simulink model "deployAMR_stateflow"  (R2024a)
settings: configuration reference "SharedConfig" (kept outside this file)
model workspace (MAT data in the model file):
  mdlWSDbList = ["C:\Users\matlab.cut\Desktop\AMR\canbus_files\tramontina_database_xsens.dbc" "tramontina_database_curtis.dbc"]
  mdlWSDbcList = ["C:\Users\rodri\Dev\Projects\External\Tramontina\atlas\interface_models\xsens.dbc" "tramontina_database_curtis.dbc"]
undefined symbols (not defined in the file): L, L_limited, magnitude, max_steering_angle_deg, num_of_wps, T, tstep, vehicle_wheelbase
libraries: simulink x3, simulink_extras x2
(part 1 of 2)
settings Model: DataDictionary=configuration_dictionary.sldd  Creator=rodri  LastModifiedBy=matlab.cut
settings ConfigSetRef: SourceName=SharedConfig

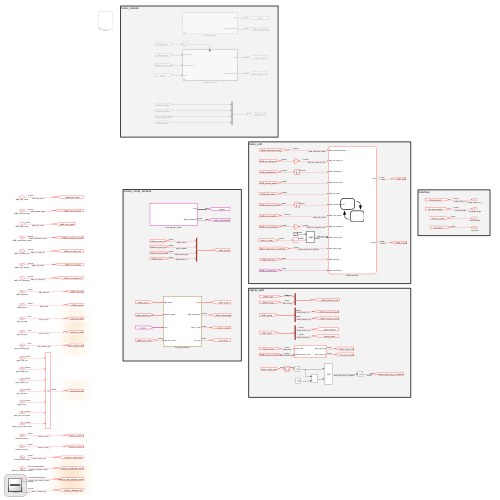
[thumbnail: Simulink's stored preview of the top-level diagram]
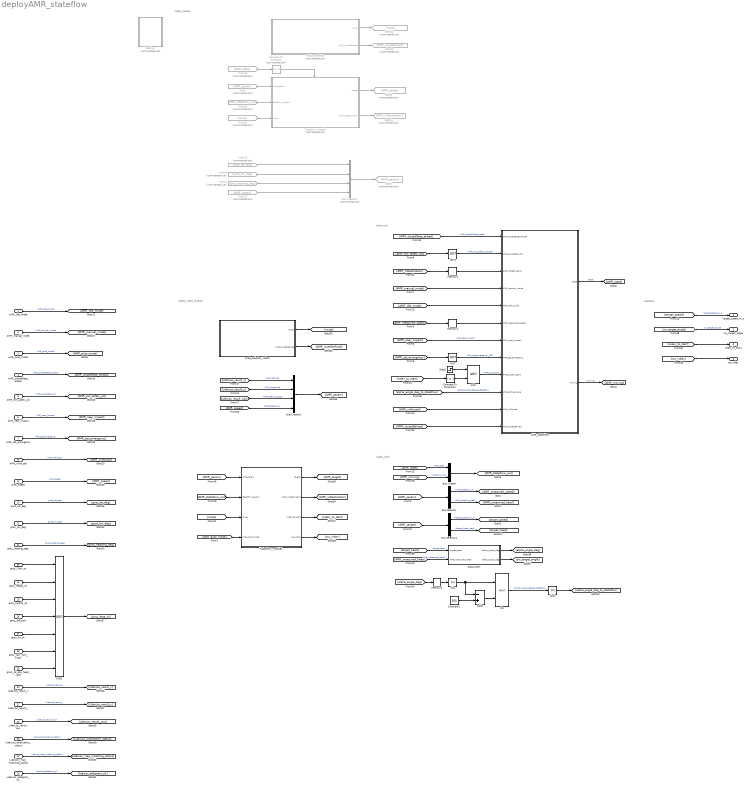
== system deployAMR_stateflow ==
  note: route_module
  note: brain_unit
  note: signal_split
  note: interface
  note: indoor_route_module
  AMR_idle_mode : Inport  OutDataTypeStr=boolean
  AMR_manual_mode : Inport  Port=2  OutDataTypeStr=boolean
  AMR_auto_mode : Inport  Port=3
  AMR_closedGate_ahead : Inport  Port=4  OutDataTypeStr=boolean
  AMR_ext_safety_plc : Inport  Port=5  OutDataTypeStr=boolean
  AMR_near_impact : Inport  Port=6  OutDataTypeStr=boolean
  AMR_set_emergency : Inport  Port=7  OutDataTypeStr=boolean
  AMR_withLoad : Inport  Port=8
  AMR_speed : Inport  Port=9
  gnss_lat_deg : Inport  Port=10  OutDataTypeStr=int32
  gnss_lon_deg : Inport  Port=11  OutDataTypeStr=int32
  gnss_heading_deg : Inport  Port=12  OutDataTypeStr=int32
  gnss_iToW_ok : Inport  Port=13
  gnss_height_ok : Inport  Port=14
  gnss_numSV_ok : Inport  Port=15
  gnss_diff_soln : Inport  Port=16
  gnss_fix_ok : Inport  Port=17
  gnss_carr_soln_fixed : Inport  Port=18
  gnss_rel_pos_head_valid : Inport  Port=19
  LidarLoc_result_x : Inport  Port=20
  LidarLoc_result_y : Inport  Port=21
  LidarLoc_result_yaw : Inport  Port=22
  LidarLoc_localization_status : Inport  Port=23  OutDataTypeStr=Enum: EnumLocalizationStatus
  LidarLoc_map_matching_status : Inport  Port=24  OutDataTypeStr=Enum: EnumMapMatchingStatus
  LidarLoc_telegram_ok : Inport  Port=25  OutDataTypeStr=boolean
  AMR_stateFlow : Stateflow chart  TreatAsAtomicUnit=on
  AND : Logic  AllPortsSameDT=off  OutDataTypeStr=boolean
  AND1 : Logic  Inputs=7  AllPortsSameDT=off  OutDataTypeStr=boolean
  Abs : Abs  SaturateOnIntegerOverflow=off
  Abs1 : Abs  SaturateOnIntegerOverflow=off
  Add1 : Sum  Inputs=-+
  Backup : Subsystem  Commented=on
  Bus Creator : BusCreator  Inputs=2
  Bus Creator1 : BusCreator  Inputs=4
  Bus Creator2 : BusCreator  Commented=on  Inputs=4
  Bus Selector : BusSelector  OutputSignals=AMR_speed_m_s,AMR_heading_deg
  Bus Selector1 : BusSelector  OutputSignals=target_speed_m_s,target_head_deg
  Compare To Constant : simulink/Logic and Bit Operations/Compare To Constant  Commented=on  relop===  const=2  OutDataTypeStr=boolean
  Compare To Constant1 : simulink/Logic and Bit Operations/Compare To Constant  relop=>=  const=1  OutDataTypeStr=boolean
  Constant2 : Constant  Value=360
  From : From  Commented=on  GotoTag=AMR_param
  From13 : From  Commented=on  GotoTag=AMR_state
  From14 : From  Commented=on  GotoTag=AMR_speed
  From18 : From  Commented=on  GotoTag=AMR_stateFlow_out
  From25 : From  Commented=on  GotoTag=route
  From29 : From  Commented=on  GotoTag=gnss_lat_deg
  From4 : From  Commented=on  GotoTag=gnss_lon_deg
  From5 : From  Commented=on  GotoTag=gnss_heading_deg
  Goto12 : Goto  Commented=on  GotoTag=route
  Goto13 : Goto  Commented=on  GotoTag=AMR_routeDefined
  Goto14 : Goto  Commented=on  GotoTag=AMR_inDestination
  Goto7 : Goto  Commented=on  GotoTag=AMR_param
  Goto8 : Goto  Commented=on  GotoTag=AMR_target
  Memory1 : Memory
  Memory2 : Memory
  Memory3 : Memory  InheritSampleTime=on
  Min : MinMax  Inputs=2
  NOT : Logic  Operator=NOT  IconShape=distinctive  AllPortsSameDT=off  OutDataTypeStr=boolean
  NOT1 : Logic  Operator=NOT  IconShape=distinctive  AllPortsSameDT=off  OutDataTypeStr=boolean
  Route_selector : Subsystem  Commented=on
  Step2 : Step  Time=10  SampleTime=0
  Subsystem : Subsystem
  Trajectory_module : Subsystem  Commented=on
  Trajectory_module1 : Subsystem
  route_selector_indoor : Subsystem
  target_speed_m_s : Outport
  sw_target_angle : Outport  Port=2
  index_to_start : Outport  Port=3
  wp_index : Outport  Port=4
  wires:
  AMR_stateFlow/2(moving) -> [AMR_moving]  "moving"
  AMR_stateFlow/1(state) -> [AMR_state]  "state"
  [AMR_ext_safety_plc] -> NOT1/1
  [AMR_manual_mode] -> AMR_stateFlow/4(AMR_manual_mode)
  [AMR_measured_speed] -> Memory1/1
  [AMR_near_impact] -> AMR_stateFlow/7(AMR_near_impact)  "AMR_near_impact"
  [AMR_set_emergency] -> NOT/1
  [AMR_withLoad] -> AMR_stateFlow/11(AMR_withLoad)
  [AMR_inDestination] -> Memory2/1
  [AMR_closedGate_ahead] -> AMR_stateFlow/1(AMR_closedGate_ahead)  "AMR_closedGate_ahead"
  From/1 -> Trajectory_module/1(AMR_param)
  Trajectory_module/1(target) -> Goto8/1
  From18/1 -> Trajectory_module/2(stateFlow_param)
  From13/1 -> Compare To Constant/1
  Compare To Constant/1 -> Trajectory_module/Enable
  [alpha_angle_deg_to_stateflow] -> AMR_stateFlow/10(AMR_alpha_angle)  "alpha_angle_deg_to_stateflow"
  Memory1/1 -> AMR_stateFlow/6(AMR_measured_speed)
  Route_selector/1(route) -> Goto12/1
  Route_selector/2(AMR_routeDefined) -> Goto13/1
  From25/1 -> Trajectory_module/3(route)
  [AMR_routeDefined] -> AMR_stateFlow/12(AMR_routeDefined)
  Trajectory_module/2(AMR_inDestination) -> Goto14/1
  Memory2/1 -> AMR_stateFlow/3(AMR_inDestination)
  AMR_closedGate_ahead/1 -> [AMR_closedGate_ahead]  "AMR_closedGate_ahead"
  AMR_manual_mode/1 -> [AMR_manual_mode]  "AMR_manual_mode"
  AMR_near_impact/1 -> [AMR_near_impact]  "AMR_near_impact"
  AMR_withLoad/1 -> [AMR_withLoad]  "AMR_withLoad"
  gnss_lat_deg/1 -> [gnss_lat_deg]  "gnss_lat_deg"
  gnss_lon_deg/1 -> [gnss_lon_deg]  "gnss_lon_deg"
  AMR_speed/1 -> [AMR_speed]  "AMR_speed"
  gnss_heading_deg/1 -> [gnss_heading_deg]  "gnss_heading_deg"
  AMR_set_emergency/1 -> [AMR_set_emergency]  "AMR_set_emergency"
  AMR_ext_safety_plc/1 -> [AMR_ext_safety_plc]  "AMR_ext_safety_plc"
  NOT1/1 -> AMR_stateFlow/2(AMR_ext_safety_plc)  "AMR_ext_safety_plc_NOT"
  NOT/1 -> AMR_stateFlow/8(AMR_set_emergency)  "AMR_set_emergency_NOT"
  Bus Creator/1 -> [AMR_stateFlow_out]
  [AMR_moving] -> Bus Creator/2  "AMR_moving"
  [AMR_state] -> Bus Creator/1  "AMR_state"
  Bus Selector/1 -> [AMR_measured_speed]  "<AMR_speed_m_s>"
  Bus Selector1/2 -> [target_head]  "<target_head_deg>"
  Bus Selector/2 -> [AMR_measured_head]  "<AMR_heading_deg>"
  Bus Selector1/1 -> [target_speed]  "<target_speed_m_s>"
  [AMR_param] -> Bus Selector/1
  [AMR_target] -> Bus Selector1/1
  [sw_target_angle] -> sw_target_angle/1  "sw_target_angle"
  [target_speed] -> target_speed_m_s/1  "target_speed_m_s"
  AMR_idle_mode/1 -> [AMR_idle_mode]  "AMR_idle_mode"
  [AMR_idle_mode] -> AMR_stateFlow/5(AMR_idle_mode)
  LidarLoc_result_x/1 -> [LidarLoc_result_x]  "LidarLoc_result_x"
  LidarLoc_result_y/1 -> [LidarLoc_result_y]  "LidarLoc_result_y"
  LidarLoc_result_yaw/1 -> [LidarLoc_result_yaw]  "LidarLoc_result_yaw"
  LidarLoc_localization_status/1 -> [LidarLoc_localization_status]  "licarLoc_licalization_status"
  LidarLoc_map_matching_status/1 -> [LidarLoc_map_matching_status]  "licarLoc_map_matching_status"
  LidarLoc_telegram_ok/1 -> [licarLoc_telegram_ok]  "licarLoc_telegram_ok"
  route_selector_indoor/2(AMR_routeDefined) -> [AMR_routeDefined]
  route_selector_indoor/1(route) -> [route]
  [route] -> Trajectory_module1/3(route)
  Trajectory_module1/1(target) -> [AMR_target]
  [AMR_param] -> Trajectory_module1/1(AMR_param)
  Bus Creator1/1 -> [AMR_param]
  [AMR_stateFlow_out] -> Trajectory_module1/2(stateFlow_param)
  Trajectory_module1/2(AMR_inDestination) -> [AMR_inDestination]
  [AMR_speed] -> Bus Creator1/4  "AMR_speed_m_s"
  [LidarLoc_result_yaw] -> Bus Creator1/3  "AMR_heading_deg"
  [LidarLoc_result_y] -> Bus Creator1/2  "AMR_Longitude"
  Bus Creator2/1 -> Goto7/1
  From29/1 -> Bus Creator2/1
  From4/1 -> Bus Creator2/2
  From5/1 -> Bus Creator2/3
  From14/1 -> Bus Creator2/4
  [LidarLoc_result_x] -> Bus Creator1/1  "AMR_Latitude"
  [AMR_measured_head] -> Subsystem/2(AMR_measured_head)  "AMR_measured_head"
  Subsystem/2(delta_angle_deg) -> [sw_target_angle]
  [target_head] -> Subsystem/1(target_head)  "target_head"
  [AMR_auto_mode] -> Trajectory_module1/4(AMR_auto_mode)
  AMR_auto_mode/1 -> [AMR_auto_mode]  "AMR_auto_mode"
  AND/1 -> AMR_stateFlow/9(AMR_system_start)  "AMR_syst_start"
  Step2/1 -> AND/1
  Compare To Constant1/1 -> AND/2
  [index_to_start] -> Compare To Constant1/1
  Trajectory_module1/3(index_to_start) -> [index_to_start]
  gnss_iToW_ok/1 -> AND1/1
  gnss_height_ok/1 -> AND1/2
  gnss_numSV_ok/1 -> AND1/3
  gnss_diff_soln/1 -> AND1/4
  AND1/1 -> [gnss_data_ok]
  gnss_fix_ok/1 -> AND1/5
  gnss_carr_soln_fixed/1 -> AND1/6
  gnss_rel_pos_head_valid/1 -> AND1/7
  Subsystem/1(alpha_angle_deg) -> [alpha_angle_deg]
  [index_to_start] -> index_to_start/1
  Trajectory_module1/4(wp_index) -> [wp_index]
  [wp_index] -> wp_index/1
  [alpha_angle_deg] -> Memory3/1
  Min/1 -> Abs1/1  "alpha_angle_deg_to_stateflow"
  Memory3/1 -> Abs/1
  Abs/1 -> Add1/1, Min/1
  Constant2/1 -> Add1/2
  Add1/1 -> Min/2
  Abs1/1 -> [alpha_angle_deg_to_stateflow]

== system deployAMR_stateflow/Backup ==
  Add : Sum  Inputs=+-
  Constant5 : Constant  Value=0
  GPS : Subsystem  Commented=on
  GPS_speed_measure : Subsystem  Commented=on
  Step : Step  Time=10  After=.000005  SampleTime=0
  Step1 : Step  Time=50  After=.000005  SampleTime=0
  wires:
  GPS_speed_measure/2(heading_deg) -> [agv_measured_heading]
  GPS/1(POS) -> [agv_pos]
  Constant5/1 -> GPS/1(dlat)
  Step1/1 -> Add/2
  Add/1 -> GPS/2(dlng)
  [agv_pos] -> GPS_speed_measure/1(GPS_POS)
  Step/1 -> Add/1
  GPS_speed_measure/1(speed_m_s) -> [agv_measured_speed]

== system deployAMR_stateflow/Route_selector ==
  Bus Creator4 : BusCreator  Inputs=2
  Constant : Constant
  Constant5 : Constant  Value=T.Latitude
  Constant9 : Constant  Value=T.Longitude
  route : Outport
  AMR_routeDefined : Outport  Port=2
  wires:
  Bus Creator4/1 -> route/1  "route"
  Constant9/1 -> Bus Creator4/2  "Longitude"
  Constant5/1 -> Bus Creator4/1  "Latitude"
  Constant/1 -> AMR_routeDefined/1

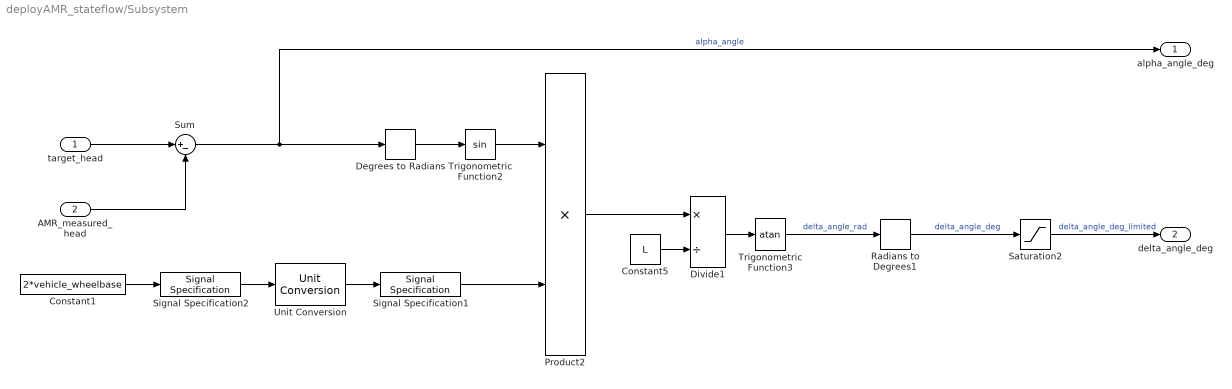
== system deployAMR_stateflow/Subsystem ==
  target_head : Inport
  AMR_measured_head : Inport  Port=2
  Constant1 : Constant  Value=2*vehicle_wheelbase
  Constant5 : Constant  Value=L
  Degrees to Radians : simulink_extras/Transformations/Degrees to Radians
  Divide1 : Product  Inputs=*/
  Product2 : Product
  Radians to Degrees1 : simulink_extras/Transformations/Radians to Degrees
  Saturation2 : Saturate  UpperLimit=max_steering_angle_deg  LowerLimit=-max_steering_angle_deg
  Signal Specification1 : SignalSpecification  Unit=m
  Signal Specification2 : SignalSpecification  Unit=mm
  Sum : Sum  Inputs=|+-
  Trigonometric Function2 : Trigonometry
  Trigonometric Function3 : Trigonometry  Operator=atan  ApproximationMethod=CORDIC
  Unit Conversion : UnitConversion
  alpha_angle_deg : Outport
  delta_angle_deg : Outport  Port=2
  wires:
  Degrees to Radians/1 -> Trigonometric Function2/1
  Constant1/1 -> Signal Specification2/1
  Product2/1 -> Divide1/1
  Radians to Degrees1/1 -> Saturation2/1  "delta_angle_deg"
  Sum/1 -> Degrees to Radians/1, alpha_angle_deg/1  "alpha_angle"
  Trigonometric Function2/1 -> Product2/1
  Constant5/1 -> Divide1/2
  Trigonometric Function3/1 -> Radians to Degrees1/1  "delta_angle_rad"
  Divide1/1 -> Trigonometric Function3/1
  target_head/1 -> Sum/1
  AMR_measured_head/1 -> Sum/2
  Saturation2/1 -> delta_angle_deg/1  "delta_angle_deg_limited"
  Unit Conversion/1 -> Signal Specification1/1
  Signal Specification2/1 -> Unit Conversion/1
  Signal Specification1/1 -> Product2/2

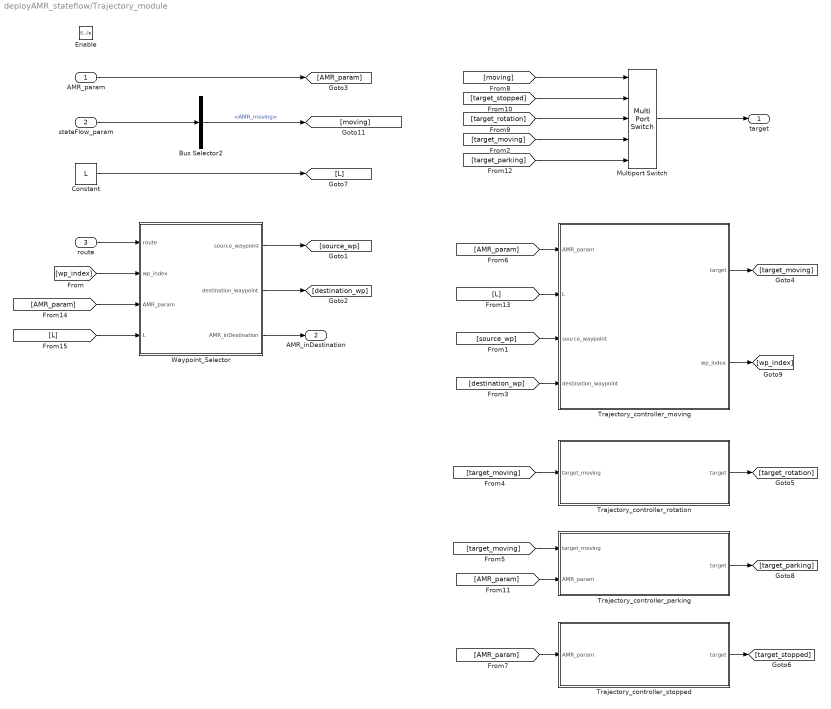
== system deployAMR_stateflow/Trajectory_module ==
  AMR_param : Inport
  stateFlow_param : Inport  Port=2
  route : Inport  Port=3
  Enable : EnablePort
  Bus Selector2 : BusSelector  OutputSignals=AMR_moving
  Constant : Constant  Value=L
  Multiport Switch : MultiPortSwitch  DataPortOrder=Zero-based contiguous  Inputs=4  zeroidx=on  SaturateOnIntegerOverflow=off  InputSameDT=off
  Trajectory_controller_moving : Subsystem
  Trajectory_controller_parking : Subsystem
  Trajectory_controller_rotation : Subsystem
  Trajectory_controller_stopped : Subsystem
  Waypoint_Selector : Subsystem
  target : Outport
  AMR_inDestination : Outport  Port=2
  wires:
  Trajectory_controller_moving/2(wp_index) -> [wp_index]
  [wp_index] -> Waypoint_Selector/2(wp_index)
  Trajectory_controller_moving/1(target) -> [target_moving]
  route/1 -> Waypoint_Selector/1(route)
  [L] -> Trajectory_controller_moving/2(L)
  Bus Selector2/1 -> [moving]  "<AMR_moving>"
  stateFlow_param/1 -> Bus Selector2/1
  [source_wp] -> Trajectory_controller_moving/3(source_waypoint)
  Waypoint_Selector/1(source_waypoint) -> [source_wp]
  Waypoint_Selector/2(destination_waypoint) -> [destination_wp]
  [destination_wp] -> Trajectory_controller_moving/4(destination_waypoint)
  AMR_param/1 -> [AMR_param]
  [AMR_param] -> Trajectory_controller_moving/1(AMR_param)
  Trajectory_controller_rotation/1(target) -> [target_rotation]
  Multiport Switch/1 -> target/1
  [moving] -> Multiport Switch/1
  [target_stopped] -> Multiport Switch/2
  [target_parking] -> Multiport Switch/5
  [target_moving] -> Multiport Switch/4
  [target_rotation] -> Multiport Switch/3
  [target_moving] -> Trajectory_controller_rotation/1(target_moving)
  [target_moving] -> Trajectory_controller_parking/1(target_moving)
  Trajectory_controller_parking/1(target) -> [target_parking]
  [AMR_param] -> Trajectory_controller_parking/2(AMR_param)
  [AMR_param] -> Trajectory_controller_stopped/1(AMR_param)
  Trajectory_controller_stopped/1(target) -> [target_stopped]
  Constant/1 -> [L]
  [AMR_param] -> Waypoint_Selector/3(AMR_param)
  [L] -> Waypoint_Selector/4(L)
  Waypoint_Selector/3(AMR_inDestination) -> AMR_inDestination/1

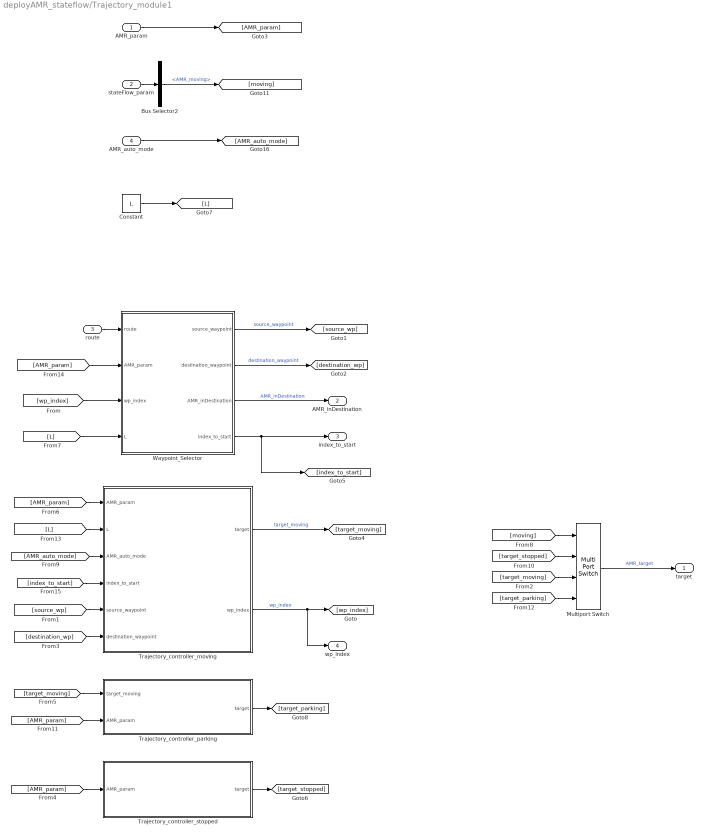
== system deployAMR_stateflow/Trajectory_module1 ==
  AMR_param : Inport
  stateFlow_param : Inport  Port=2
  route : Inport  Port=3
  AMR_auto_mode : Inport  Port=4
  Bus Selector2 : BusSelector  OutputSignals=AMR_moving
  Constant : Constant  Value=L
  Multiport Switch : MultiPortSwitch  DataPortOrder=Zero-based contiguous  zeroidx=on  SaturateOnIntegerOverflow=off  InputSameDT=off
  Trajectory_controller_moving : Subsystem
  Trajectory_controller_parking : Subsystem
  Trajectory_controller_stopped : Subsystem
  Waypoint_Selector : Subsystem
  target : Outport
  AMR_inDestination : Outport  Port=2
  index_to_start : Outport  Port=3
  wp_index : Outport  Port=4
  wires:
  Trajectory_controller_moving/2(wp_index) -> wp_index/1, [wp_index]  "wp_index"
  [wp_index] -> Waypoint_Selector/3(wp_index)
  Trajectory_controller_moving/1(target) -> [target_moving]  "target_moving"
  route/1 -> Waypoint_Selector/1(route)
  [L] -> Trajectory_controller_moving/2(L)
  Bus Selector2/1 -> [moving]  "<AMR_moving>"
  stateFlow_param/1 -> Bus Selector2/1
  [source_wp] -> Trajectory_controller_moving/5(source_waypoint)
  Waypoint_Selector/1(source_waypoint) -> [source_wp]  "source_waypoint"
  Waypoint_Selector/2(destination_waypoint) -> [destination_wp]  "destination_waypoint"
  [destination_wp] -> Trajectory_controller_moving/6(destination_waypoint)
  AMR_param/1 -> [AMR_param]
  [AMR_param] -> Trajectory_controller_moving/1(AMR_param)
  Multiport Switch/1 -> target/1  "AMR_target"
  [moving] -> Multiport Switch/1
  [target_stopped] -> Multiport Switch/2
  [target_moving] -> Trajectory_controller_parking/1(target_moving)
  Trajectory_controller_parking/1(target) -> [target_parking]
  [AMR_param] -> Trajectory_controller_parking/2(AMR_param)
  [AMR_param] -> Trajectory_controller_stopped/1(AMR_param)
  Trajectory_controller_stopped/1(target) -> [target_stopped]
  Constant/1 -> [L]
  [AMR_param] -> Waypoint_Selector/2(AMR_param)
  [L] -> Waypoint_Selector/4(L)
  Waypoint_Selector/3(AMR_inDestination) -> AMR_inDestination/1  "AMR_inDestination"
  [target_moving] -> Multiport Switch/3
  [target_parking] -> Multiport Switch/4
  AMR_auto_mode/1 -> [AMR_auto_mode]
  [AMR_auto_mode] -> Trajectory_controller_moving/3(AMR_auto_mode)
  [index_to_start] -> Trajectory_controller_moving/4(index_to_start)
  Waypoint_Selector/4(index_to_start) -> [index_to_start], index_to_start/1

== system deployAMR_stateflow/route_selector_indoor ==
  Bus Creator : BusCreator  Inputs=2
  Constant : Constant  Value=T.X
  Constant1 : Constant  Value=T.Y
  Constant2 : Constant
  route : Outport
  AMR_routeDefined : Outport  Port=2
  wires:
  Constant1/1 -> Bus Creator/2  "Y"
  Constant/1 -> Bus Creator/1  "X"
  Bus Creator/1 -> route/1  "route"
  Constant2/1 -> AMR_routeDefined/1

== system deployAMR_stateflow/Backup/GPS ==
  dlat : Inport
  dlng : Inport  Port=2
  Add : Sum  Inputs=|++
  Add1 : Sum  Inputs=|++
  Matrix Concatenate : Concatenate  Mode=Multidimensional array  ConcatenateDimension=2
  lat : Memory  InitialCondition=-29.272334
  lng : Memory  InitialCondition=-51.467679
  POS : Outport
  wires:
  lat/1 -> Add1/2, Matrix Concatenate/1
  Matrix Concatenate/1 -> POS/1
  dlat/1 -> Add1/1
  Add1/1 -> lat/1
  lng/1 -> Add/2, Matrix Concatenate/2
  Add/1 -> lng/1
  dlng/1 -> Add/1

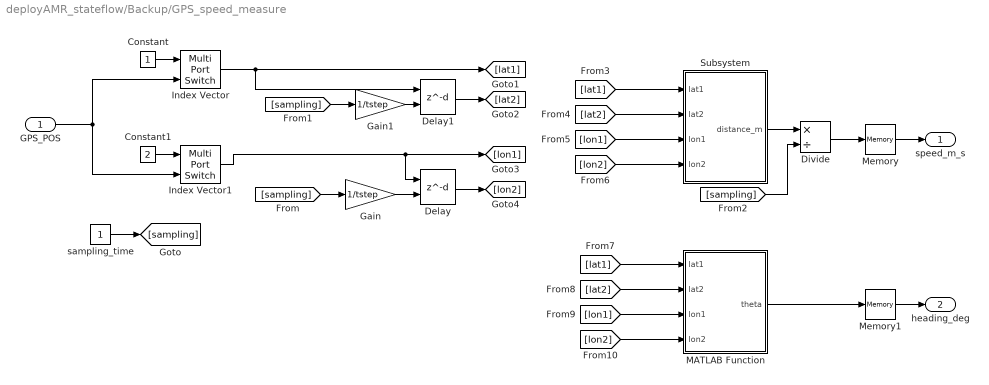
== system deployAMR_stateflow/Backup/GPS_speed_measure ==
  GPS_POS : Inport
  Constant : Constant
  Constant1 : Constant  Value=2
  Delay : Delay  DelayLengthSource=Input port  DelayLength=5/tstep  InitialCondition=-51.467679
      settings: InputPortMap=u0,p1
  Delay1 : Delay  DelayLengthSource=Input port  DelayLength=5/tstep  InitialCondition=-29.272334
      settings: InputPortMap=u0,p1
  Divide : Product  Inputs=*/
  Gain : Gain  Gain=1/tstep
  Gain1 : Gain  Gain=1/tstep
  Index Vector : MultiPortSwitch  Inputs=1  SaturateOnIntegerOverflow=off  InputSameDT=off
  Index Vector1 : MultiPortSwitch  Inputs=1  SaturateOnIntegerOverflow=off  InputSameDT=off
  MATLAB Function : MATLAB Function  TreatAsAtomicUnit=on
  Memory : Memory
  Memory1 : Memory
  Subsystem : Subsystem
  sampling_time : Constant
  speed_m_s : Outport
  heading_deg : Outport  Port=2
  wires:
  Subsystem/1(distance_m) -> Divide/1
  Memory/1 -> speed_m_s/1
  Divide/1 -> Memory/1
  Constant/1 -> Index Vector/1
  Constant1/1 -> Index Vector1/1
  Index Vector1/1 -> [lon1], Delay/1
  sampling_time/1 -> [sampling]
  Gain/1 -> Delay/2
  [sampling] -> Gain/1
  [sampling] -> Gain1/1
  Gain1/1 -> Delay1/2
  Index Vector/1 -> [lat1], Delay1/1
  GPS_POS/1 -> Index Vector/2, Index Vector1/2
  [sampling] -> Divide/2
  Memory1/1 -> heading_deg/1
  Delay1/1 -> [lat2]
  Delay/1 -> [lon2]
  [lat2] -> Subsystem/2(lat2)
  [lon1] -> Subsystem/3(lon1)
  [lon2] -> Subsystem/4(lon2)
  [lat1] -> Subsystem/1(lat1)
  [lon2] -> MATLAB Function/4(lon2)
  [lat1] -> MATLAB Function/1(lat1)
  [lon1] -> MATLAB Function/3(lon1)
  [lat2] -> MATLAB Function/2(lat2)
  MATLAB Function/1(theta) -> Memory1/1

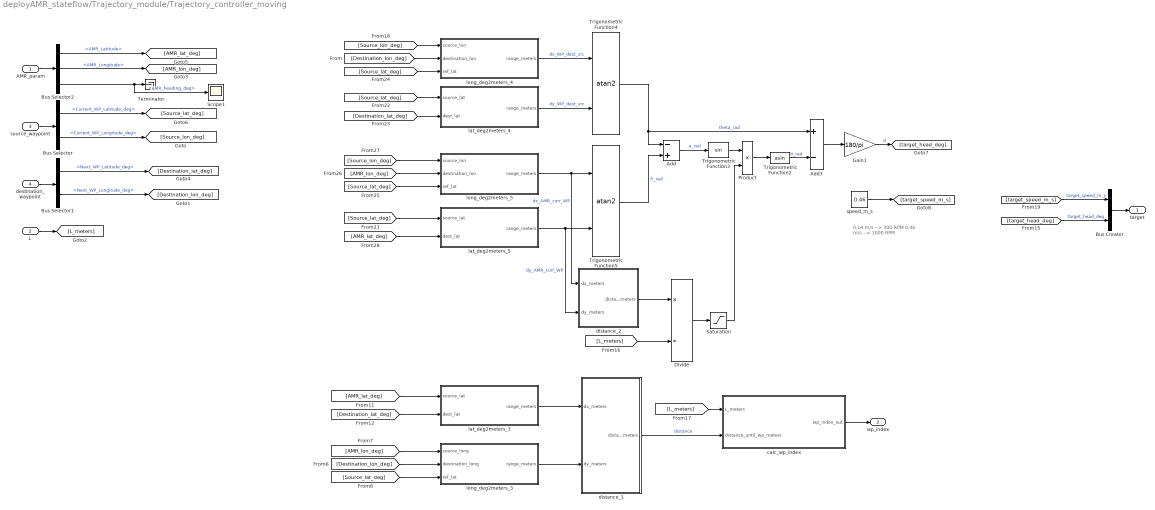
== system deployAMR_stateflow/Trajectory_module/Trajectory_controller_moving ==
  note: 0.14 m/s --> 300 RPM
      | 0.46 m/s --> 1000 RPM
  AMR_param : Inport
  L : Inport  Port=2
  source_waypoint : Inport  Port=3
  destination_waypoint : Inport  Port=4
  Add : Sum  Inputs=-+
  Add3 : Sum  Inputs=+-
  Bus Creator : BusCreator  Inputs=2
  Bus Selector : BusSelector  OutputSignals=Current_WP_Latitude_deg,Current_WP_Longitude_deg
  Bus Selector1 : BusSelector  OutputSignals=Next_WP_Latitude_deg,Next_WP_Longitude_deg
  Bus Selector2 : BusSelector  OutputSignals=AMR_Latitude,AMR_Longitude,AMR_heading_deg
  Divide : Product  Inputs=*/
  Gain1 : Gain  Gain=180/pi
  Product : Product
  Saturation : Saturate  UpperLimit=1  LowerLimit=0
  Scope1 : Scope
  Terminator : Terminator
  Trigonometric Function2 : Trigonometry  Operator=asin
  Trigonometric Function3 : Trigonometry
  Trigonometric Function4 : Trigonometry  Operator=atan2
  Trigonometric Function5 : Trigonometry  Operator=atan2
  calc_wp_index : Subsystem
  distance_1 : Subsystem  TreatAsAtomicUnit=on
  distance_2 : Subsystem  TreatAsAtomicUnit=on
  lat_deg2meters_3 : Subsystem  TreatAsAtomicUnit=on
  lat_deg2meters_4 : Subsystem  TreatAsAtomicUnit=on
  lat_deg2meters_5 : Subsystem  TreatAsAtomicUnit=on
  long_deg2meters_3 : Subsystem  TreatAsAtomicUnit=on
  long_deg2meters_4 : Subsystem  TreatAsAtomicUnit=on
  long_deg2meters_5 : Subsystem  TreatAsAtomicUnit=on
  speed_m_s : Constant  Value=0.46
  target : Outport
  wp_index : Outport  Port=2
  wires:
  distance_1/1(distance_meters) -> calc_wp_index/2(distance_until_wp_meters)  "distance"
  calc_wp_index/1(wp_index_out) -> wp_index/1
  [Destination_lon_deg] -> long_deg2meters_3/2(destination_long)
  [Source_lat_deg] -> long_deg2meters_3/3(ref_lat)
  Trigonometric Function4/1 -> Add3/1, Add/1  "theta_rad"
  [L_meters] -> Divide/2
  [L_meters] -> calc_wp_index/1(L_meters)
  source_waypoint/1 -> Bus Selector/1
  destination_waypoint/1 -> Bus Selector1/1
  AMR_param/1 -> Bus Selector2/1
  Bus Selector2/1 -> [AMR_lat_deg]  "<AMR_Latitude>"
  Bus Selector2/2 -> [AMR_lon_deg]  "<AMR_Longitude>"
  Bus Selector/1 -> [Source_lat_deg]  "<Current_WP_Latitude_deg>"
  Bus Selector1/2 -> [Destination_lon_deg]  "<Next_WP_Longitude_deg>"
  Bus Selector1/1 -> [Destination_lat_deg]  "<Next_WP_Latitude_deg>"
  Bus Selector/2 -> [Source_lon_deg]  "<Current_WP_Longitude_deg>"
  [AMR_lon_deg] -> long_deg2meters_3/1(source_long)
  L/1 -> [L_meters]
  [target_speed_m_s] -> Bus Creator/1  "target_speed_m_s"
  [target_head_deg] -> Bus Creator/2  "target_head_deg"
  Bus Creator/1 -> target/1
  Add/1 -> Trigonometric Function3/1  "a_rad"
  Trigonometric Function3/1 -> Product/1
  speed_m_s/1 -> [target_speed_m_s]
  Bus Selector2/3 -> Scope1/1, Terminator/1  "<AMR_heading_deg>"
  Gain1/1 -> [target_head_deg]  "d"
  distance_2/1(distance_meters) -> Divide/1
  [Destination_lat_deg] -> lat_deg2meters_3/2(dest_lat)
  [AMR_lat_deg] -> lat_deg2meters_3/1(source_lat)
  Trigonometric Function5/1 -> Add/2  "fi_rad"
  lat_deg2meters_3/1(range_meters) -> distance_1/1(dx_meters)
  long_deg2meters_3/1(range_meters) -> distance_1/2(dy_meters)
  long_deg2meters_4/1(range_meters) -> Trigonometric Function4/1  "dx_WP_dest_src"
  lat_deg2meters_4/1(range_meters) -> Trigonometric Function4/2  "dy_WP_dest_src"
  long_deg2meters_5/1(range_meters) -> distance_2/1(dx_meters), Trigonometric Function5/1  "dx_AMR_curr_WP"
  lat_deg2meters_5/1(range_meters) -> distance_2/2(dy_meters), Trigonometric Function5/2  "dy_AMR_curr_WP"
  Add3/1 -> Gain1/1
  [Source_lon_deg] -> long_deg2meters_5/1(source_lon)
  [Source_lat_deg] -> long_deg2meters_4/3(ref_lat)
  [Source_lat_deg] -> lat_deg2meters_4/1(source_lat)
  [Destination_lon_deg] -> long_deg2meters_4/2(destination_lon)
  [AMR_lon_deg] -> long_deg2meters_5/2(destination_lon)
  [Source_lat_deg] -> long_deg2meters_5/3(ref_lat)
  [Destination_lat_deg] -> lat_deg2meters_4/2(dest_lat)
  [Source_lat_deg] -> lat_deg2meters_5/1(source_lat)
  [Source_lon_deg] -> long_deg2meters_4/1(source_lon)
  [AMR_lat_deg] -> lat_deg2meters_5/2(dest_lat)
  Trigonometric Function2/1 -> Add3/2  "b_rad"
  Product/1 -> Trigonometric Function2/1
  Divide/1 -> Saturation/1
  Saturation/1 -> Product/2

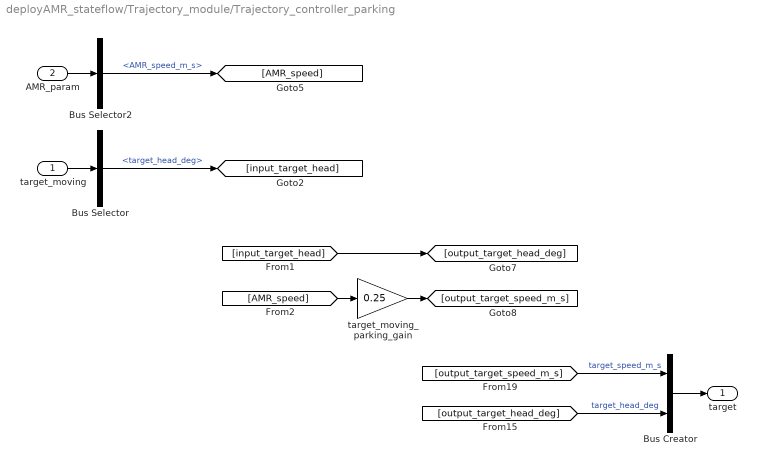
== system deployAMR_stateflow/Trajectory_module/Trajectory_controller_parking ==
  target_moving : Inport
  AMR_param : Inport  Port=2
  Bus Creator : BusCreator  Inputs=2
  Bus Selector : BusSelector  OutputSignals=target_head_deg
  Bus Selector2 : BusSelector  OutputSignals=AMR_speed_m_s
  target_moving_parking_gain : Gain  Gain=0.25
  target : Outport
  wires:
  [output_target_speed_m_s] -> Bus Creator/1  "target_speed_m_s"
  [output_target_head_deg] -> Bus Creator/2  "target_head_deg"
  Bus Creator/1 -> target/1
  [input_target_head] -> [output_target_head_deg]
  target_moving/1 -> Bus Selector/1
  AMR_param/1 -> Bus Selector2/1
  Bus Selector2/1 -> [AMR_speed]  "<AMR_speed_m_s>"
  Bus Selector/1 -> [input_target_head]  "<target_head_deg>"
  target_moving_parking_gain/1 -> [output_target_speed_m_s]
  [AMR_speed] -> target_moving_parking_gain/1

== system deployAMR_stateflow/Trajectory_module/Trajectory_controller_rotation ==
  target_moving : Inport
  Bus Creator : BusCreator  Inputs=2
  Bus Selector : BusSelector  OutputSignals=target_speed_m_s,target_head_deg
  target_moving_rotation_gain : Gain  Gain=0.5
  target : Outport
  wires:
  [output_target_speed_m_s] -> Bus Creator/1  "target_speed_m_s"
  [output_target_head_deg] -> Bus Creator/2  "target_head_deg"
  Bus Creator/1 -> target/1
  target_moving/1 -> Bus Selector/1
  Bus Selector/1 -> [input_target_speed]  "<target_speed_m_s>"
  Bus Selector/2 -> [input_target_head]  "<target_head_deg>"
  [input_target_speed] -> target_moving_rotation_gain/1
  [input_target_head] -> [output_target_head_deg]
  target_moving_rotation_gain/1 -> [output_target_speed_m_s]

== system deployAMR_stateflow/Trajectory_module/Trajectory_controller_stopped ==
  AMR_param : Inport
  Bus Creator : BusCreator  Inputs=2
  Bus Selector2 : BusSelector  OutputSignals=AMR_heading_deg
  Constant : Constant  Value=0
  target : Outport
  wires:
  [output_target_speed_m_s] -> Bus Creator/1  "target_speed_m_s"
  [output_target_head_deg] -> Bus Creator/2  "target_head_deg"
  Bus Creator/1 -> target/1
  [AMR_head] -> [output_target_head_deg]
  AMR_param/1 -> Bus Selector2/1
  Bus Selector2/1 -> [AMR_head]  "<AMR_heading_deg>"
  Constant/1 -> [output_target_speed_m_s]

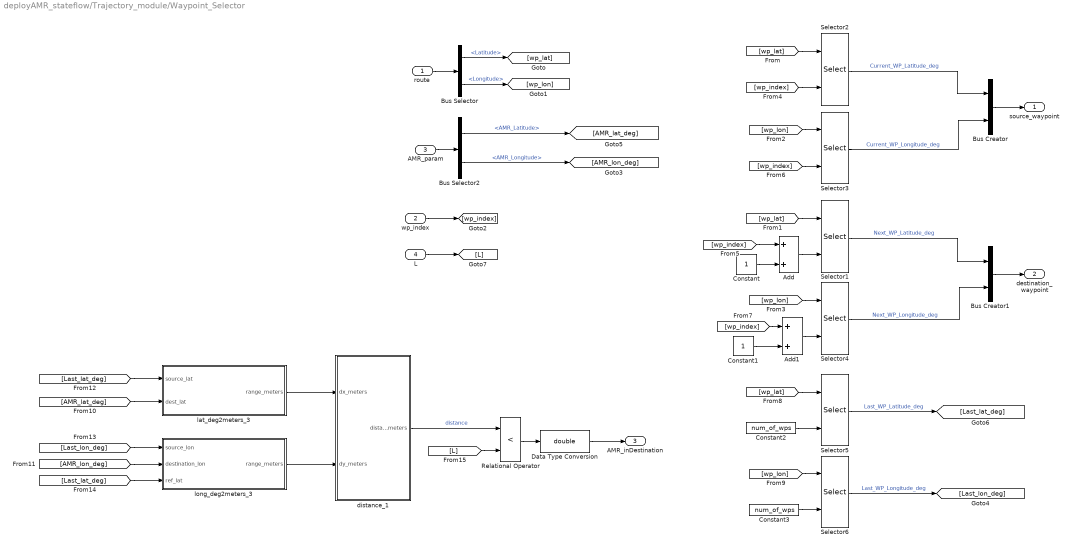
== system deployAMR_stateflow/Trajectory_module/Waypoint_Selector ==
  route : Inport
  wp_index : Inport  Port=2
  AMR_param : Inport  Port=3
  L : Inport  Port=4
  Add : Sum
  Add1 : Sum
  Bus Creator : BusCreator  Inputs=2
  Bus Creator1 : BusCreator  Inputs=2
  Bus Selector : BusSelector  OutputSignals=Latitude,Longitude
  Bus Selector2 : BusSelector  OutputSignals=AMR_Latitude,AMR_Longitude
  Constant : Constant
  Constant1 : Constant
  Constant2 : Constant  Value=num_of_wps
  Constant3 : Constant  Value=num_of_wps
  Data Type Conversion : DataTypeConversion  OutDataTypeStr=double  SaturateOnIntegerOverflow=off  RndMeth=Floor
  Relational Operator : RelationalOperator  Operator=<  OutDataTypeStr=boolean  RndMeth=Simplest  InputSameDT=off
  Selector{1..6} (6 alike) : Selector  InputPortWidth=num_of_wps  IndexOptions=Index vector (port)  Indices=[1 3]  OutputSizes=1
  distance_1 : Subsystem  TreatAsAtomicUnit=on
  lat_deg2meters_3 : Subsystem  TreatAsAtomicUnit=on
  long_deg2meters_3 : Subsystem  TreatAsAtomicUnit=on
  source_waypoint : Outport
  destination_waypoint : Outport  Port=2
  AMR_inDestination : Outport  Port=3
  wires:
  Selector2/1 -> Bus Creator/1  "Current_WP_Latitude_deg"
  Add/1 -> Selector1/2
  Constant/1 -> Add/2
  Constant1/1 -> Add1/2
  Add1/1 -> Selector4/2
  route/1 -> Bus Selector/1
  Bus Selector/1 -> [wp_lat]  "<Latitude>"
  Bus Selector/2 -> [wp_lon]  "<Longitude>"
  [wp_lat] -> Selector2/1
  [wp_lat] -> Selector1/1
  [wp_lon] -> Selector3/1
  [wp_lon] -> Selector4/1
  wp_index/1 -> [wp_index]
  [wp_index] -> Selector2/2
  [wp_index] -> Add/1
  [wp_index] -> Selector3/2
  [wp_index] -> Add1/1
  Bus Creator/1 -> source_waypoint/1
  Selector3/1 -> Bus Creator/2  "Current_WP_Longitude_deg"
  Selector4/1 -> Bus Creator1/2  "Next_WP_Longitude_deg"
  Selector1/1 -> Bus Creator1/1  "Next_WP_Latitude_deg"
  Bus Creator1/1 -> destination_waypoint/1
  Bus Selector2/1 -> [AMR_lat_deg]  "<AMR_Latitude>"
  AMR_param/1 -> Bus Selector2/1
  Bus Selector2/2 -> [AMR_lon_deg]  "<AMR_Longitude>"
  [wp_lat] -> Selector5/1
  [wp_lon] -> Selector6/1
  Constant3/1 -> Selector6/2
  Constant2/1 -> Selector5/2
  long_deg2meters_3/1(range_meters) -> distance_1/2(dy_meters)
  lat_deg2meters_3/1(range_meters) -> distance_1/1(dx_meters)
  Selector5/1 -> [Last_lat_deg]  "Last_WP_Latitude_deg"
  Selector6/1 -> [Last_lon_deg]  "Last_WP_Longitude_deg"
  [Last_lat_deg] -> lat_deg2meters_3/1(source_lat)
  [Last_lon_deg] -> long_deg2meters_3/1(source_lon)
  [Last_lat_deg] -> long_deg2meters_3/3(ref_lat)
  [AMR_lat_deg] -> lat_deg2meters_3/2(dest_lat)
  [AMR_lon_deg] -> long_deg2meters_3/2(destination_lon)
  Relational Operator/1 -> Data Type Conversion/1
  distance_1/1(distance_meters) -> Relational Operator/1  "distance"
  L/1 -> [L]
  [L] -> Relational Operator/2
  Data Type Conversion/1 -> AMR_inDestination/1

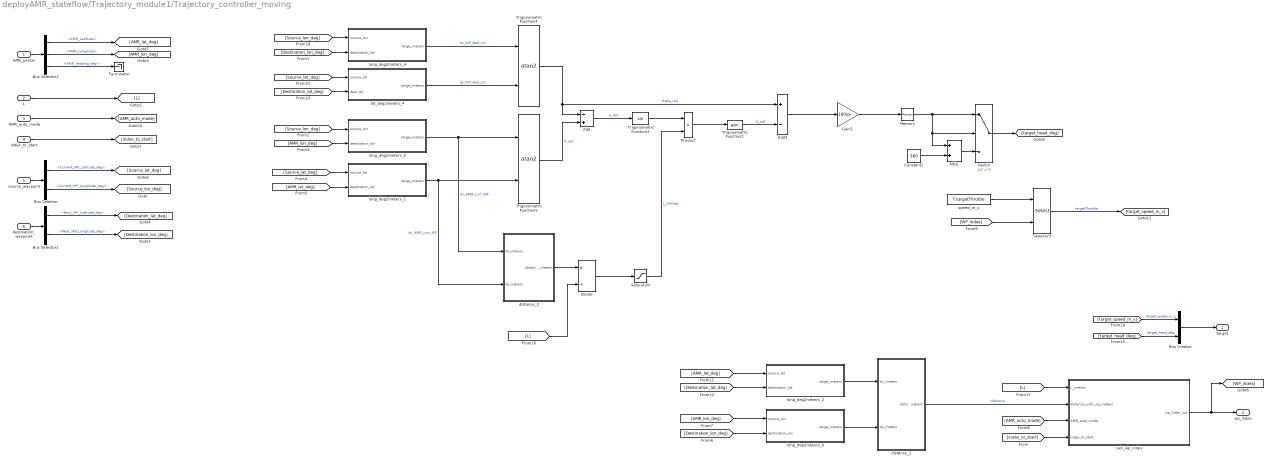
== system deployAMR_stateflow/Trajectory_module1/Trajectory_controller_moving ==
  AMR_param : Inport
  L : Inport  Port=2
  AMR_auto_mode : Inport  Port=3
  index_to_start : Inport  Port=4
  source_waypoint : Inport  Port=5
  destination_waypoint : Inport  Port=6
  Add : Sum  Inputs=-+
  Add1 : Sum
  Add3 : Sum  Inputs=+-
  Bus Creator : BusCreator  Inputs=2
  Bus Selector : BusSelector  OutputSignals=Current_WP_Latitude_deg,Current_WP_Longitude_deg
  Bus Selector1 : BusSelector  OutputSignals=Next_WP_Latitude_deg,Next_WP_Longitude_deg
  Bus Selector2 : BusSelector  OutputSignals=AMR_Latitude,AMR_Longitude,AMR_heading_deg
  Constant2 : Constant  Value=360
  Divide : Product  Inputs=*/
  Gain1 : Gain  Gain=180/pi
  Memory : Memory  InitialCondition=T.Yaw(1)  InheritSampleTime=on
  Product : Product
  Saturation : Saturate  UpperLimit=L_limited  LowerLimit=0
  Selector3 : Selector  InputPortWidth=num_of_wps  IndexOptions=Index vector (port)  Indices=[1 3]  OutputSizes=1
  Switch : Switch  Criteria=u2 > Threshold  SaturateOnIntegerOverflow=off  InputSameDT=off
  Terminator : Terminator
  Trigonometric Function2 : Trigonometry  Operator=asin
  Trigonometric Function3 : Trigonometry
  Trigonometric Function4 : Trigonometry  Operator=atan2
  Trigonometric Function5 : Trigonometry  Operator=atan2
  calc_wp_index : Subsystem
  distance_1 : Subsystem  TreatAsAtomicUnit=on
  distance_2 : Subsystem  TreatAsAtomicUnit=on
  lat_deg2meters_4 : Subsystem  TreatAsAtomicUnit=on
  long_deg2meters_1 : Subsystem  TreatAsAtomicUnit=on
  long_deg2meters_2 : Subsystem  TreatAsAtomicUnit=on
  long_deg2meters_4 : Subsystem  TreatAsAtomicUnit=on
  long_deg2meters_5 : Subsystem  TreatAsAtomicUnit=on
  long_deg2meters_6 : Subsystem  TreatAsAtomicUnit=on
  speed_m_s : Constant  Value=T.targetThrottle
  target : Outport
  wp_index : Outport  Port=2
  wires:
  [Source_lon_deg] -> long_deg2meters_5/1(source_lon)
  Add/1 -> Trigonometric Function3/1  "a_rad"
  [Destination_lat_deg] -> lat_deg2meters_4/2(dest_lat)
  Switch/1 -> [target_head_deg]
  distance_2/1(distance_meters) -> Divide/1
  Saturation/1 -> Product/2  "L_limited"
  Add1/1 -> Switch/3
  Product/1 -> Trigonometric Function2/1
  [AMR_lon_deg] -> long_deg2meters_5/2(destination_lon)
  Bus Creator/1 -> target/1
  destination_waypoint/1 -> Bus Selector1/1
  Add3/1 -> Gain1/1
  long_deg2meters_5/1(range_meters) -> Trigonometric Function5/1, distance_2/1(dx_meters)  "dx_AMR_curr_WP"
  [L] -> Divide/2
  AMR_param/1 -> Bus Selector2/1
  [Source_lon_deg] -> long_deg2meters_4/1(source_lon)
  lat_deg2meters_4/1(range_meters) -> Trigonometric Function4/2  "dy_WP_dest_src"
  [Destination_lat_deg] -> long_deg2meters_2/2(destination_lat)
  [Source_lat_deg] -> lat_deg2meters_4/1(source_lat)
  [AMR_lat_deg] -> long_deg2meters_2/1(source_lat)
  Trigonometric Function3/1 -> Product/1
  L/1 -> [L]
  Bus Selector2/3 -> Terminator/1  "<AMR_heading_deg>"
  long_deg2meters_2/1(range_meters) -> distance_1/1(dx_meters)
  [target_head_deg] -> Bus Creator/2  "target_head_deg"
  [Destination_lon_deg] -> long_deg2meters_6/2(destination_lon)
  Trigonometric Function5/1 -> Add/2  "fi_rad"
  Bus Selector2/1 -> [AMR_lat_deg]  "<AMR_Latitude>"
  Divide/1 -> Saturation/1
  Bus Selector2/2 -> [AMR_lon_deg]  "<AMR_Longitude>"
  Bus Selector/1 -> [Source_lat_deg]  "<Current_WP_Latitude_deg>"
  long_deg2meters_4/1(range_meters) -> Trigonometric Function4/1  "dx_WP_dest_src"
  [Destination_lon_deg] -> long_deg2meters_4/2(destination_lon)
  [Source_lat_deg] -> long_deg2meters_1/1(source_lat)
  [target_speed_m_s] -> Bus Creator/1  "target_speed_m_s"
  [AMR_lon_deg] -> long_deg2meters_6/1(source_lon)
  [AMR_lat_deg] -> long_deg2meters_1/2(destination_lat)
  Bus Selector1/1 -> [Destination_lat_deg]  "<Next_WP_Latitude_deg>"
  source_waypoint/1 -> Bus Selector/1
  Trigonometric Function4/1 -> Add3/1, Add/1  "theta_rad"
  Bus Selector1/2 -> [Destination_lon_deg]  "<Next_WP_Longitude_deg>"
  [L] -> calc_wp_index/1(L_meters)
  long_deg2meters_1/1(range_meters) -> Trigonometric Function5/2, distance_2/2(dy_meters)  "dy_AMR_curr_WP"
  Trigonometric Function2/1 -> Add3/2  "b_rad"
  long_deg2meters_6/1(range_meters) -> distance_1/2(dy_meters)
  Bus Selector/2 -> [Source_lon_deg]  "<Current_WP_Longitude_deg>"
  Constant2/1 -> Add1/2
  Gain1/1 -> Memory/1
  [AMR_auto_mode] -> calc_wp_index/3(AMR_auto_mode)
  [index_to_start] -> calc_wp_index/4(index_to_start)
  index_to_start/1 -> [index_to_start]
  AMR_auto_mode/1 -> [AMR_auto_mode]
  distance_1/1(distance_meters) -> calc_wp_index/2(distance_until_wp_meters)  "distance"
  [WP_index] -> Selector3/2
  Selector3/1 -> [target_speed_m_s]  "targetThrottle"
  speed_m_s/1 -> Selector3/1
  calc_wp_index/1(wp_index_out) -> [WP_index], wp_index/1
  Memory/1 -> Add1/1, Switch/2, Switch/1

== system deployAMR_stateflow/Trajectory_module1/Trajectory_controller_parking ==
  target_moving : Inport
  AMR_param : Inport  Port=2
  Bus Creator : BusCreator  Inputs=2
  Bus Selector : BusSelector  OutputSignals=target_head_deg
  Bus Selector2 : BusSelector  OutputSignals=AMR_speed_m_s
  Gain : Gain  Gain=0
  target : Outport
  wires:
  [output_target_speed_m_s] -> Bus Creator/1  "target_speed_m_s"
  [output_target_head_deg] -> Bus Creator/2  "target_head_deg"
  Bus Creator/1 -> target/1
  [input_target_head] -> [output_target_head_deg]
  target_moving/1 -> Bus Selector/1
  AMR_param/1 -> Bus Selector2/1
  Bus Selector2/1 -> [AMR_speed]  "<AMR_speed_m_s>"
  Bus Selector/1 -> [input_target_head]  "<target_head_deg>"
  Gain/1 -> [output_target_speed_m_s]
  [AMR_speed] -> Gain/1

== system deployAMR_stateflow/Trajectory_module1/Trajectory_controller_stopped ==
  AMR_param : Inport
  Bus Creator : BusCreator  Inputs=2
  Bus Selector2 : BusSelector  OutputSignals=AMR_heading_deg
  Constant : Constant  Value=0
  target : Outport
  wires:
  [output_target_speed_m_s] -> Bus Creator/1  "target_speed_m_s"
  [output_target_head_deg] -> Bus Creator/2  "target_head_deg"
  Bus Creator/1 -> target/1
  [AMR_head] -> [output_target_head_deg]
  AMR_param/1 -> Bus Selector2/1
  Bus Selector2/1 -> [AMR_head]  "<AMR_heading_deg>"
  Constant/1 -> [output_target_speed_m_s]

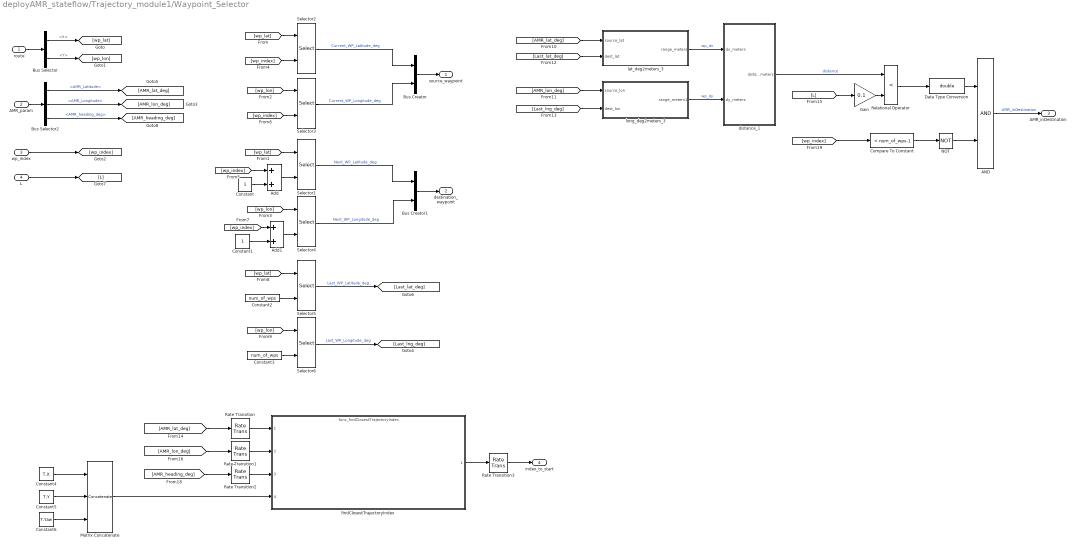
== system deployAMR_stateflow/Trajectory_module1/Waypoint_Selector ==
  route : Inport
  AMR_param : Inport  Port=2
  wp_index : Inport  Port=3
  L : Inport  Port=4
  AND : Logic  AllPortsSameDT=off  OutDataTypeStr=boolean
  Add : Sum
  Add1 : Sum
  Bus Creator : BusCreator  Inputs=2
  Bus Creator1 : BusCreator  Inputs=2
  Bus Selector : BusSelector  OutputSignals=X,Y
  Bus Selector2 : BusSelector  OutputSignals=AMR_Latitude,AMR_Longitude,AMR_heading_deg
  Compare To Constant : simulink/Logic and Bit Operations/Compare To Constant  relop=<  const=num_of_wps-1  OutDataTypeStr=boolean
  Constant : Constant
  Constant1 : Constant
  Constant2 : Constant  Value=num_of_wps
  Constant3 : Constant  Value=num_of_wps
  Constant4 : Constant  Value=T.X
  Constant5 : Constant  Value=T.Y
  Constant6 : Constant  Value=T.Yaw
  Data Type Conversion : DataTypeConversion  OutDataTypeStr=double  SaturateOnIntegerOverflow=off  RndMeth=Floor
  Gain : Gain  Gain=0.1
  Matrix Concatenate : Concatenate  NumInputs=3  Mode=Multidimensional array  ConcatenateDimension=2
  NOT : Logic  Operator=NOT  IconShape=distinctive  AllPortsSameDT=off  OutDataTypeStr=boolean
  Rate Transition{,1..3} (4 alike) : RateTransition
  Relational Operator : RelationalOperator  Operator=<  OutDataTypeStr=boolean  RndMeth=Simplest  InputSameDT=off
  Selector{1..6} (6 alike) : Selector  InputPortWidth=num_of_wps  IndexOptions=Index vector (port)  Indices=[1 3]  OutputSizes=1
  distance_1 : Subsystem  TreatAsAtomicUnit=on
  findClosestTrajectoryIndex : ModelReference  ModelNameDialog=func_findClosestTrajectoryIndex.slx  SimulationMode=Normal  ModelReferenceVersion=1.242
  lat_deg2meters_3 : Subsystem  TreatAsAtomicUnit=on
  long_deg2meters_3 : Subsystem  TreatAsAtomicUnit=on
  source_waypoint : Outport
  destination_waypoint : Outport  Port=2
  AMR_inDestination : Outport  Port=3
  index_to_start : Outport  Port=4
  wires:
  Selector2/1 -> Bus Creator/1  "Current_WP_Latitude_deg"
  Add/1 -> Selector1/2
  Constant/1 -> Add/2
  Constant1/1 -> Add1/2
  Add1/1 -> Selector4/2
  route/1 -> Bus Selector/1
  Bus Selector/1 -> [wp_lat]  "<X>"
  Bus Selector/2 -> [wp_lon]  "<Y>"
  [wp_lat] -> Selector2/1
  [wp_lat] -> Selector1/1
  [wp_lon] -> Selector3/1
  [wp_lon] -> Selector4/1
  wp_index/1 -> [wp_index]
  [wp_index] -> Selector2/2
  [wp_index] -> Add/1
  [wp_index] -> Selector3/2
  [wp_index] -> Add1/1
  Bus Creator/1 -> source_waypoint/1
  Selector3/1 -> Bus Creator/2  "Current_WP_Longitude_deg"
  Selector4/1 -> Bus Creator1/2  "Next_WP_Longitude_deg"
  Selector1/1 -> Bus Creator1/1  "Next_WP_Latitude_deg"
  Bus Creator1/1 -> destination_waypoint/1
  Bus Selector2/1 -> [AMR_lat_deg]  "<AMR_Latitude>"
  AMR_param/1 -> Bus Selector2/1
  Bus Selector2/2 -> [AMR_lon_deg]  "<AMR_Longitude>"
  [wp_lat] -> Selector5/1
  [wp_lon] -> Selector6/1
  Constant3/1 -> Selector6/2
  Constant2/1 -> Selector5/2
  long_deg2meters_3/1(range_meters1) -> distance_1/2(dy_meters)  "wp_dy"
  lat_deg2meters_3/1(range_meters) -> distance_1/1(dx_meters)  "wp_dx"
  Selector5/1 -> [Last_lat_deg]  "Last_WP_Latitude_deg"
  Selector6/1 -> [Last_lng_deg]  "Last_WP_Longitude_deg"
  [AMR_lat_deg] -> lat_deg2meters_3/1(source_lat)
  Relational Operator/1 -> Data Type Conversion/1
  distance_1/1(distance_meters) -> Relational Operator/1  "distance"
  L/1 -> [L]
  [L] -> Gain/1
  Data Type Conversion/1 -> AND/1
  [Last_lat_deg] -> lat_deg2meters_3/2(dest_lat)
  [AMR_lon_deg] -> long_deg2meters_3/1(source_lon)
  [Last_lng_deg] -> long_deg2meters_3/2(dest_lon)
  Matrix Concatenate/1 -> findClosestTrajectoryIndex/4
  [AMR_heading_deg] -> Rate Transition2/1
  [AMR_lon_deg] -> Rate Transition1/1
  Constant6/1 -> Matrix Concatenate/3
  Constant4/1 -> Matrix Concatenate/1
  [AMR_lat_deg] -> Rate Transition/1
  Constant5/1 -> Matrix Concatenate/2
  Bus Selector2/3 -> [AMR_heading_deg]  "<AMR_heading_deg>"
  findClosestTrajectoryIndex/1 -> Rate Transition3/1
  Rate Transition/1 -> findClosestTrajectoryIndex/1
  Rate Transition1/1 -> findClosestTrajectoryIndex/2
  Rate Transition2/1 -> findClosestTrajectoryIndex/3
  Rate Transition3/1 -> index_to_start/1
  [wp_index] -> Compare To Constant/1
  Compare To Constant/1 -> NOT/1
  NOT/1 -> AND/2
  AND/1 -> AMR_inDestination/1  "AMR_inDestination"
  Gain/1 -> Relational Operator/2

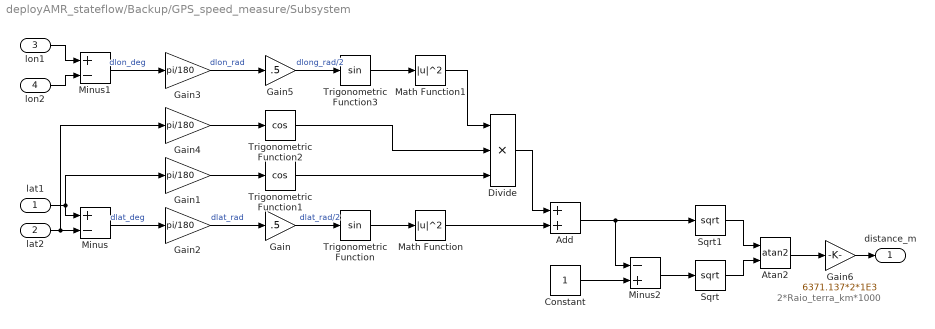
== system deployAMR_stateflow/Backup/GPS_speed_measure/Subsystem ==
  note: 2*Raio_terra_km*1000
  lat1 : Inport
  lat2 : Inport  Port=2
  lon1 : Inport  Port=3
  lon2 : Inport  Port=4
  Add : Sum
  Atan2 : Trigonometry  Operator=atan2
  Constant : Constant
  Divide : Product  Inputs=***
  Gain : Gain  Gain=.5
  Gain{1..4} (4 alike) : Gain  Gain=pi/180
  Gain5 : Gain  Gain=.5
  Gain6 : Gain  Gain=6371.137*2*1E3
  Math Function : Math  Operator=magnitude^2
  Math Function1 : Math  Operator=magnitude^2
  Minus : Sum  Inputs=+-
  Minus1 : Sum  Inputs=+-
  Minus2 : Sum  Inputs=-+
  Sqrt : Sqrt
  Sqrt1 : Sqrt
  Trigonometric Function : Trigonometry
  Trigonometric Function1 : Trigonometry  Operator=cos
  Trigonometric Function2 : Trigonometry  Operator=cos
  Trigonometric Function3 : Trigonometry
  distance_m : Outport
  wires:
  Minus/1 -> Gain2/1  "dlat_deg"
  Minus1/1 -> Gain3/1  "dlon_deg"
  lat2/1 -> Gain4/1, Minus/2
  lat1/1 -> Gain1/1, Minus/1
  lon1/1 -> Minus1/1
  lon2/1 -> Minus1/2
  Gain2/1 -> Gain/1  "dlat_rad"
  Gain/1 -> Trigonometric Function/1  "dlat_rad/2"
  Trigonometric Function/1 -> Math Function/1
  Math Function/1 -> Add/2
  Gain1/1 -> Trigonometric Function1/1
  Gain4/1 -> Trigonometric Function2/1
  Divide/1 -> Add/1
  Trigonometric Function3/1 -> Math Function1/1
  Gain5/1 -> Trigonometric Function3/1  "dlong_rad/2"
  Gain3/1 -> Gain5/1  "dlon_rad"
  Trigonometric Function1/1 -> Divide/3
  Trigonometric Function2/1 -> Divide/2
  Math Function1/1 -> Divide/1
  Add/1 -> Minus2/1, Sqrt1/1
  Minus2/1 -> Sqrt/1
  Atan2/1 -> Gain6/1
  Gain6/1 -> distance_m/1
  Constant/1 -> Minus2/2
  Sqrt1/1 -> Atan2/1
  Sqrt/1 -> Atan2/2

== system deployAMR_stateflow/Trajectory_module/Trajectory_controller_moving/calc_wp_index ==
  L_meters : Inport
  distance_until_wp_meters : Inport  Port=2
  Add : Sum
  Constant : Constant
  Data Type Conversion : DataTypeConversion  OutDataTypeStr=double  SaturateOnIntegerOverflow=off  RndMeth=Floor
  Memory : Memory  InitialCondition=1
  Relational Operator : RelationalOperator  Operator=>  OutDataTypeStr=boolean  RndMeth=Simplest  InputSameDT=off
  Saturation : Saturate  UpperLimit=num_of_wps-1  LowerLimit=1
  Scope3 : Scope
  Switch : Switch  Criteria=u2 > Threshold  Threshold=.5  SaturateOnIntegerOverflow=off  InputSameDT=off
  wp_index_out : Outport
  wires:
  distance_until_wp_meters/1 -> Relational Operator/1
  L_meters/1 -> Relational Operator/2
  Relational Operator/1 -> Data Type Conversion/1
  Data Type Conversion/1 -> Switch/2
  Switch/1 -> Memory/1
  Add/1 -> Switch/3
  Constant/1 -> Add/1
  [WP_index] -> wp_index_out/1, Scope3/1
  [WP_index] -> Switch/1
  [WP_index] -> Add/2
  Saturation/1 -> [WP_index]
  Memory/1 -> Saturation/1

== system deployAMR_stateflow/Trajectory_module/Trajectory_controller_moving/distance_1 ==
  dx_meters : Inport
  dy_meters : Inport  Port=2
  Add : Sum
  Divide1 : Product  Inputs=**
  Divide2 : Product  Inputs=**
  Sqrt : Sqrt
  distance_meters : Outport
  wires:
  dx_meters/1 -> Divide1/2, Divide1/1
  Divide1/1 -> Add/1
  Add/1 -> Sqrt/1
  dy_meters/1 -> Divide2/2, Divide2/1
  Divide2/1 -> Add/2
  Sqrt/1 -> distance_meters/1

== system deployAMR_stateflow/Trajectory_module/Trajectory_controller_moving/distance_2 ==
  dx_meters : Inport
  dy_meters : Inport  Port=2
  Add : Sum
  Divide1 : Product  Inputs=**
  Divide2 : Product  Inputs=**
  Sqrt : Sqrt
  distance_meters : Outport
  wires:
  dx_meters/1 -> Divide1/2, Divide1/1
  Divide1/1 -> Add/1
  Add/1 -> Sqrt/1
  dy_meters/1 -> Divide2/2, Divide2/1
  Divide2/1 -> Add/2
  Sqrt/1 -> distance_meters/1

== system deployAMR_stateflow/Trajectory_module/Trajectory_controller_moving/lat_deg2meters_3 ==
  source_lat : Inport
  dest_lat : Inport  Port=2
  Add : Sum  Inputs=+-
  deg2meters : Gain  Gain=111195
  range_meters : Outport
  wires:
  Add/1 -> deg2meters/1
  deg2meters/1 -> range_meters/1
  dest_lat/1 -> Add/1
  source_lat/1 -> Add/2

== system deployAMR_stateflow/Trajectory_module/Trajectory_controller_moving/lat_deg2meters_4 ==
  source_lat : Inport
  dest_lat : Inport  Port=2
  Add : Sum  Inputs=+-
  deg2meters : Gain  Gain=111195
  range_meters : Outport
  wires:
  Add/1 -> deg2meters/1
  deg2meters/1 -> range_meters/1
  dest_lat/1 -> Add/1
  source_lat/1 -> Add/2

== system deployAMR_stateflow/Trajectory_module/Trajectory_controller_moving/lat_deg2meters_5 ==
  source_lat : Inport
  dest_lat : Inport  Port=2
  Add : Sum  Inputs=+-
  deg2meters : Gain  Gain=111195
  range_meters : Outport
  wires:
  Add/1 -> deg2meters/1
  deg2meters/1 -> range_meters/1
  dest_lat/1 -> Add/1
  source_lat/1 -> Add/2

== system deployAMR_stateflow/Trajectory_module/Trajectory_controller_moving/long_deg2meters_3 ==
  source_long : Inport
  destination_long : Inport  Port=2
  ref_lat : Inport  Port=3
  Add : Sum  Inputs=+-
  Constant : Constant  Value=1E-4
  Divide : Product  Inputs=**
  Switch : Switch  Criteria=u2 ~= 0  SaturateOnIntegerOverflow=off  InputSameDT=off
  Trigonometric Function2 : Trigonometry  Operator=cos
  deg2meters : Gain  Gain=111195
  deg2rad : Gain  Gain=pi/180
  range_meters : Outport
  wires:
  Trigonometric Function2/1 -> Divide/2
  deg2rad/1 -> Trigonometric Function2/1
  ref_lat/1 -> deg2rad/1
  Constant/1 -> Switch/3
  source_long/1 -> Add/2
  Add/1 -> deg2meters/1
  deg2meters/1 -> Divide/1
  Switch/1 -> range_meters/1
  destination_long/1 -> Add/1
  Divide/1 -> Switch/2, Switch/1

== system deployAMR_stateflow/Trajectory_module/Trajectory_controller_moving/long_deg2meters_4 ==
  source_lon : Inport
  destination_lon : Inport  Port=2
  ref_lat : Inport  Port=3
  Add : Sum  Inputs=+-
  Divide : Product  Inputs=**
  Trigonometric Function2 : Trigonometry  Operator=cos
  deg2meters : Gain  Gain=111195
  deg2rad : Gain  Gain=pi/180
  range_meters : Outport
  wires:
  Trigonometric Function2/1 -> Divide/2
  deg2rad/1 -> Trigonometric Function2/1
  ref_lat/1 -> deg2rad/1
  source_lon/1 -> Add/2
  Add/1 -> deg2meters/1
  deg2meters/1 -> Divide/1
  Divide/1 -> range_meters/1
  destination_lon/1 -> Add/1

== system deployAMR_stateflow/Trajectory_module/Trajectory_controller_moving/long_deg2meters_5 ==
  source_lon : Inport
  destination_lon : Inport  Port=2
  ref_lat : Inport  Port=3
  Add : Sum  Inputs=+-
  Divide : Product  Inputs=**
  Trigonometric Function2 : Trigonometry  Operator=cos
  deg2meters : Gain  Gain=111195
  deg2rad : Gain  Gain=pi/180
  range_meters : Outport
  wires:
  Trigonometric Function2/1 -> Divide/2
  deg2rad/1 -> Trigonometric Function2/1
  ref_lat/1 -> deg2rad/1
  source_lon/1 -> Add/2
  Add/1 -> deg2meters/1
  deg2meters/1 -> Divide/1
  destination_lon/1 -> Add/1
  Divide/1 -> range_meters/1

== system deployAMR_stateflow/Trajectory_module/Waypoint_Selector/distance_1 ==
  dx_meters : Inport
  dy_meters : Inport  Port=2
  Add : Sum
  Divide1 : Product  Inputs=**
  Divide2 : Product  Inputs=**
  Sqrt : Sqrt
  distance_meters : Outport
  wires:
  dx_meters/1 -> Divide1/2, Divide1/1
  Divide1/1 -> Add/1
  Add/1 -> Sqrt/1
  dy_meters/1 -> Divide2/2, Divide2/1
  Divide2/1 -> Add/2
  Sqrt/1 -> distance_meters/1

== system deployAMR_stateflow/Trajectory_module/Waypoint_Selector/lat_deg2meters_3 ==
  source_lat : Inport
  dest_lat : Inport  Port=2
  Add : Sum  Inputs=+-
  deg2meters : Gain  Gain=111195
  range_meters : Outport
  wires:
  Add/1 -> deg2meters/1
  deg2meters/1 -> range_meters/1
  dest_lat/1 -> Add/1
  source_lat/1 -> Add/2

== system deployAMR_stateflow/Trajectory_module/Waypoint_Selector/long_deg2meters_3 ==
  source_lon : Inport
  destination_lon : Inport  Port=2
  ref_lat : Inport  Port=3
  Add : Sum  Inputs=+-
  Constant : Constant  Value=1E-4
  Divide : Product  Inputs=**
  Switch : Switch  Criteria=u2 ~= 0  SaturateOnIntegerOverflow=off  InputSameDT=off
  Trigonometric Function2 : Trigonometry  Operator=cos
  deg2meters : Gain  Gain=111195
  deg2rad : Gain  Gain=pi/180
  range_meters : Outport
  wires:
  Trigonometric Function2/1 -> Divide/2
  deg2rad/1 -> Trigonometric Function2/1
  ref_lat/1 -> deg2rad/1
  Constant/1 -> Switch/3
  source_lon/1 -> Add/2
  Add/1 -> deg2meters/1
  deg2meters/1 -> Divide/1
  Switch/1 -> range_meters/1
  destination_lon/1 -> Add/1
  Divide/1 -> Switch/2, Switch/1

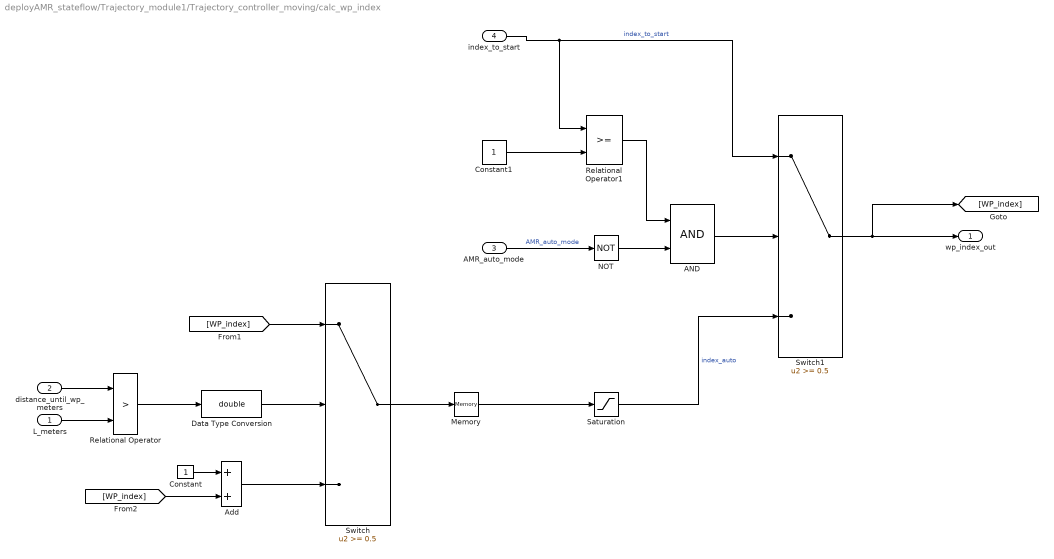
== system deployAMR_stateflow/Trajectory_module1/Trajectory_controller_moving/calc_wp_index ==
  L_meters : Inport
  distance_until_wp_meters : Inport  Port=2
  AMR_auto_mode : Inport  Port=3
  index_to_start : Inport  Port=4
  AND : Logic  AllPortsSameDT=off  OutDataTypeStr=boolean
  Add : Sum
  Constant : Constant
  Constant1 : Constant
  Data Type Conversion : DataTypeConversion  OutDataTypeStr=double  SaturateOnIntegerOverflow=off  RndMeth=Floor
  Memory : Memory  InitialCondition=1
  NOT : Logic  Operator=NOT  IconShape=distinctive  AllPortsSameDT=off  OutDataTypeStr=boolean
  Relational Operator : RelationalOperator  Operator=>  OutDataTypeStr=boolean  RndMeth=Simplest  InputSameDT=off
  Relational Operator1 : RelationalOperator  OutDataTypeStr=boolean  RndMeth=Simplest  InputSameDT=off
  Saturation : Saturate  UpperLimit=num_of_wps-1  LowerLimit=1
  Switch : Switch  Threshold=0.5  SaturateOnIntegerOverflow=off  InputSameDT=off
  Switch1 : Switch  Threshold=0.5  SaturateOnIntegerOverflow=off  InputSameDT=off
  wp_index_out : Outport
  wires:
  NOT/1 -> AND/2
  AND/1 -> Switch1/2
  AMR_auto_mode/1 -> NOT/1  "AMR_auto_mode"
  Relational Operator1/1 -> AND/1
  Constant1/1 -> Relational Operator1/2
  index_to_start/1 -> Relational Operator1/1, Switch1/1  "index_to_start"
  Saturation/1 -> Switch1/3  "index_auto"
  Switch1/1 -> wp_index_out/1, [WP_index]
  Memory/1 -> Saturation/1
  [WP_index] -> Add/2
  [WP_index] -> Switch/1
  Constant/1 -> Add/1
  Add/1 -> Switch/3
  Switch/1 -> Memory/1
  Data Type Conversion/1 -> Switch/2
  Relational Operator/1 -> Data Type Conversion/1
  L_meters/1 -> Relational Operator/2
  distance_until_wp_meters/1 -> Relational Operator/1

== system deployAMR_stateflow/Trajectory_module1/Trajectory_controller_moving/distance_1 ==
  dx_meters : Inport
  dy_meters : Inport  Port=2
  Add : Sum
  Divide1 : Product  Inputs=**
  Divide2 : Product  Inputs=**
  Sqrt : Sqrt
  distance_meters : Outport
  wires:
  dx_meters/1 -> Divide1/2, Divide1/1
  Divide1/1 -> Add/1
  Add/1 -> Sqrt/1
  dy_meters/1 -> Divide2/2, Divide2/1
  Divide2/1 -> Add/2
  Sqrt/1 -> distance_meters/1

== system deployAMR_stateflow/Trajectory_module1/Trajectory_controller_moving/distance_2 ==
  dx_meters : Inport
  dy_meters : Inport  Port=2
  Add : Sum
  Divide1 : Product  Inputs=**
  Divide2 : Product  Inputs=**
  Sqrt : Sqrt
  distance_meters : Outport
  wires:
  dx_meters/1 -> Divide1/2, Divide1/1
  Divide1/1 -> Add/1
  Add/1 -> Sqrt/1
  dy_meters/1 -> Divide2/2, Divide2/1
  Divide2/1 -> Add/2
  Sqrt/1 -> distance_meters/1

== system deployAMR_stateflow/Trajectory_module1/Trajectory_controller_moving/lat_deg2meters_4 ==
  source_lat : Inport
  dest_lat : Inport  Port=2
  Add : Sum  Inputs=+-
  range_meters : Outport
  wires:
  Add/1 -> range_meters/1
  dest_lat/1 -> Add/1
  source_lat/1 -> Add/2

== system deployAMR_stateflow/Trajectory_module1/Trajectory_controller_moving/long_deg2meters_1 ==
  source_lat : Inport
  destination_lat : Inport  Port=2
  Add : Sum  Inputs=+-
  range_meters : Outport
  wires:
  source_lat/1 -> Add/2
  destination_lat/1 -> Add/1
  Add/1 -> range_meters/1
